simulink model "sampleModel84"  (R2021b)
settings: Solver=VariableStepAuto  StartTime=0.0  StopTime=10.0  RelTol=1e-3
undefined symbols (not defined in the file or in its folder): DiscIntNeverNeededParam, Newton, Raphson
libraries: simulink x7
settings Model: Creator=user  LastModifiedBy=user

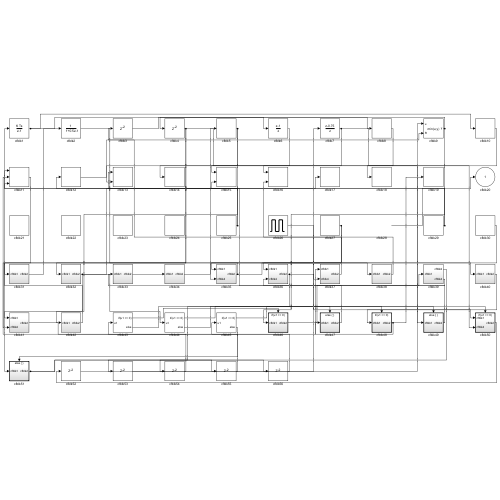
[thumbnail: Simulink's stored preview of the top-level diagram]
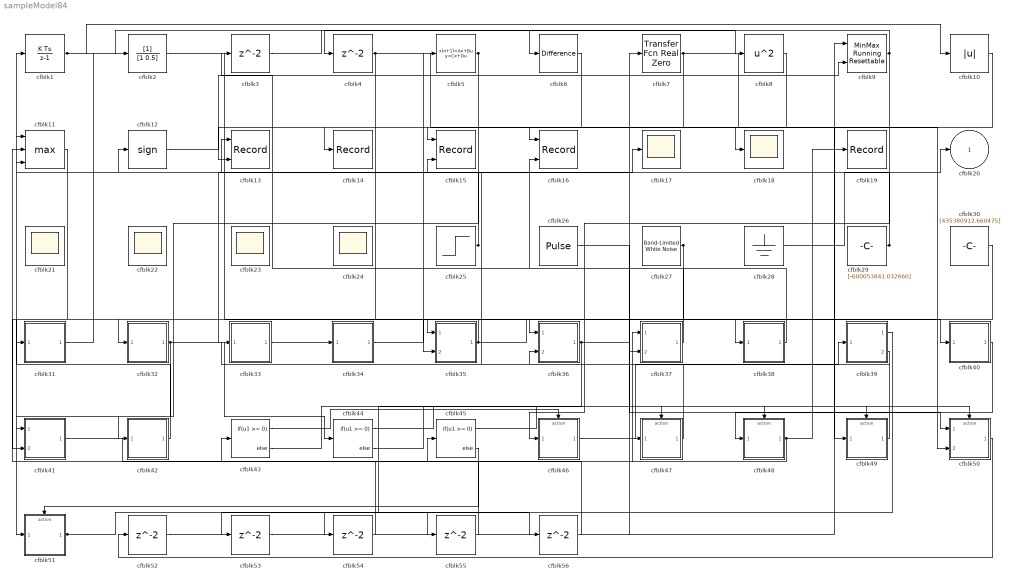
== system sampleModel84 ==
  cfblk1 : DiscreteIntegrator  ICPrevOutput=DiscIntNeverNeededParam  ICPrevScaledInput=DiscIntNeverNeededParam
  cfblk10 : Abs
  cfblk11 : MinMax  Function=max  Inputs=3
  cfblk12 : Signum
  cfblk13 : Record  FileSettingsInternal="{\"entries\":[{\"content\":{\"excelSettings\":{\"content\":{},\"type\":\"Streamout.ExcelSettings\"}},\"type\":\"Streamout.FileSettingStorage\",\"uuid\":\"6d5ab0e1-b9df-4df2-b804-9cd61c6ebc61\"}],\"packageUris\":[\"http://schema.mathworks.com/mf0/streamout_blocks/R2020a\"],\"version\":\"1.0\"}"  Layout=[1 1]  SignalsInternal="{\"entries\":[{\"content\":{\"signals\":[{\"content\":{\"blockPath\":[\"sampleModel84/cfblk13\"],\"channel\":[],\"dimensions\":[1],\"domain\":\"sampleModel84/cfblk13\",\"lineColor\":\"#a2142f\",\"plots\":[1],\"port\":1,\"sid\":[\"\"],\"signalID\":3042,\"signalName\":\"cfblk25\"},\"type\":\"RecordBlkView.Signal\",\"uuid\":\"d763d9ff-3473-40db-b6f0-cc00d4cb158e\"},{\"content\":{\"blockPath\":[\"sampleModel84/cfblk13\"],\"channel\":[],\"dimensions\":[1],\"domain\":\"sampleModel84/cfblk13\",\"lineColor\":\"#139fff\",\"plots\":[1],\"port\":2,\"sid\":[\"\"],\"signalID\":3046,\"signalName\":\"cfblk7\"},\"type\":\"RecordBlkView.Signal\",\"uuid\":\"d27f5f61-b032-4120-a613-3f0224b6e019\"}]},\"type\":\"RecordBlkView.InputSignals\",\"uuid\":\"3bd982ab-766d-439c-941a-6008472352c4\"}],\"packageUris\":[\"http://schema.mathworks.com/mf0/streamout_blocks/R2020a\"],\"version\":\"1.0\"}"  VisualizationBindings="{\"xyplotplugin\":{\"info\":[{\"series\":[{\"bindingParametersList\":[{\"parameter\":\"X-Axis\",\"signalID\":3042,\"signalName\":\"cfblk25\"},{\"parameter\":\"Y-Axis\",\"signalID\":3046,\"signalName\":\"cfblk7\"}],\"seriesID\":61716}],\"subplotID\":1}]}}"  CompatibilityTag=XY
  cfblk14 : Record  FileSettingsInternal="{\"entries\":[{\"content\":{\"excelSettings\":{\"content\":{},\"type\":\"Streamout.ExcelSettings\"}},\"type\":\"Streamout.FileSettingStorage\",\"uuid\":\"01d03471-c07e-448c-bcd4-e8026727b8ae\"}],\"packageUris\":[\"http://schema.mathworks.com/mf0/streamout_blocks/R2020a\"],\"version\":\"1.0\"}"  SignalsInternal="{\"entries\":[{\"content\":{\"signals\":[{\"content\":{\"blockPath\":[\"sampleModel84/cfblk14\"],\"channel\":[],\"dimensions\":[1],\"domain\":\"sampleModel84/cfblk14\",\"lineColor\":\"#a2142f\",\"plots\":[1],\"port\":1,\"sid\":[\"\"],\"signalID\":3050,\"signalName\":\"cfblk8\"},\"type\":\"RecordBlkView.Signal\",\"uuid\":\"eb13109a-bc49-49c4-8163-c11cf7b14920\"}]},\"type\":\"RecordBlkView.InputSignals\",\"uuid\":\"b3fcaa82-4256-42bf-8fc9-15e04aac9106\"}],\"packageUris\":[\"http://schema.mathworks.com/mf0/streamout_blocks/R2020a\"],\"version\":\"1.0\"}"  VisualizationBindings="{\"sparklinesplugin\":{\"info\":[{\"bindingParametersList\":[],\"subplotID\":1}]}}"
  cfblk15 : Record  FileSettingsInternal="{\"entries\":[{\"content\":{\"excelSettings\":{\"content\":{},\"type\":\"Streamout.ExcelSettings\"}},\"type\":\"Streamout.FileSettingStorage\",\"uuid\":\"8215706d-99e3-4ed1-b040-388dff8976c3\"}],\"packageUris\":[\"http://schema.mathworks.com/mf0/streamout_blocks/R2020a\"],\"version\":\"1.0\"}"  Layout=[1 1]  SignalsInternal="{\"entries\":[{\"content\":{\"signals\":[{\"content\":{\"blockPath\":[\"sampleModel84/cfblk15\"],\"channel\":[],\"dimensions\":[1],\"domain\":\"sampleModel84/cfblk15\",\"lineColor\":\"#a2142f\",\"plots\":[1],\"port\":1,\"sid\":[\"\"],\"signalID\":3054,\"signalName\":\"cfblk5\"},\"type\":\"RecordBlkView.Signal\",\"uuid\":\"c065fa96-9f8c-4313-8d4b-0e94634b5292\"},{\"content\":{\"blockPath\":[\"sampleModel84/cfblk15\"],\"channel\":[],\"dimensions\":[1],\"domain\":\"sampleModel84/cfblk15\",\"lineColor\":\"#139fff\",\"plots\":[1],\"port\":2,\"sid\":[\"\"],\"signalID\":3058,\"signalName\":\"cfblk49\"},\"type\":\"RecordBlkView.Signal\",\"uuid\":\"e4297feb-6ddb-4099-b980-2a59c267fa88\"}]},\"type\":\"RecordBlkView.InputSignals\",\"uuid\":\"14db0384-847c-431a-93a3-ba0fa706bc9d\"}],\"packageUris\":[\"http://schema.mathworks.com/mf0/streamout_blocks/R2020a\"],\"version\":\"1.0\"}"  VisualizationBindings="{\"xyplotplugin\":{\"info\":[{\"series\":[{\"bindingParametersList\":[{\"parameter\":\"X-Axis\",\"signalID\":3054,\"signalName\":\"cfblk5\"},{\"parameter\":\"Y-Axis\",\"signalID\":3058,\"signalName\":\"cfblk49\"}],\"seriesID\":40958}],\"subplotID\":1}]}}"  CompatibilityTag=XY
  cfblk16 : Record  FileSettingsInternal="{\"entries\":[{\"content\":{\"excelSettings\":{\"content\":{},\"type\":\"Streamout.ExcelSettings\"}},\"type\":\"Streamout.FileSettingStorage\",\"uuid\":\"8432e45c-109e-4b5d-958a-7ed43e91799e\"}],\"packageUris\":[\"http://schema.mathworks.com/mf0/streamout_blocks/R2020a\"],\"version\":\"1.0\"}"  Layout=[1 1]  SignalsInternal="{\"entries\":[{\"content\":{\"signals\":[{\"content\":{\"blockPath\":[\"sampleModel84/cfblk16\"],\"channel\":[],\"dimensions\":[1,1],\"domain\":\"sampleModel84/cfblk16\",\"lineColor\":\"#a2142f\",\"plots\":[1],\"port\":1,\"sid\":[\"\"],\"signalID\":3062,\"signalName\":\"cfblk6\"},\"type\":\"RecordBlkView.Signal\",\"uuid\":\"d31e46d2-4c50-47c9-b63a-65829e50d0df\"},{\"content\":{\"blockPath\":[\"sampleModel84/cfblk16\"],\"channel\":[],\"dimensions\":[1],\"domain\":\"sampleModel84/cfblk16\",\"lineColor\":\"#139fff\",\"plots\":[1],\"port\":2,\"sid\":[\"\"],\"signalID\":3066,\"signalName\":\"cfblk38\"},\"type\":\"RecordBlkView.Signal\",\"uuid\":\"c6a5d8c1-6799-48d2-840e-423a328fe3fe\"}]},\"type\":\"RecordBlkView.InputSignals\",\"uuid\":\"be483031-cf2c-4130-aa2f-949f5dc1496d\"}],\"packageUris\":[\"http://schema.mathworks.com/mf0/streamout_blocks/R2020a\"],\"version\":\"1.0\"}"  VisualizationBindings="{\"xyplotplugin\":{\"info\":[{\"series\":[{\"bindingParametersList\":[{\"parameter\":\"X-Axis\",\"signalID\":3062,\"signalName\":\"cfblk6\"},{\"parameter\":\"Y-Axis\",\"signalID\":3066,\"signalName\":\"cfblk38\"}],\"seriesID\":55547}],\"subplotID\":1}]}}"  CompatibilityTag=XY
  cfblk{17..18,21..24} (6 alike) : Scope
      cfblk21 settings: Floating=on
      cfblk22 settings: Floating=on
      cfblk23 settings: Floating=on
      cfblk24 settings: Floating=on
  cfblk19 : Record  FileSettingsInternal="{\"entries\":[{\"content\":{\"excelSettings\":{\"content\":{},\"type\":\"Streamout.ExcelSettings\"}},\"type\":\"Streamout.FileSettingStorage\",\"uuid\":\"b58bf4fe-9a4f-4d8d-a211-cbcb210b0c43\"}],\"packageUris\":[\"http://schema.mathworks.com/mf0/streamout_blocks/R2020a\"],\"version\":\"1.0\"}"  SignalsInternal="{\"entries\":[{\"content\":{\"signals\":[{\"content\":{\"blockPath\":[\"sampleModel84/cfblk19\"],\"channel\":[],\"dimensions\":[1,1],\"domain\":\"sampleModel84/cfblk19\",\"lineColor\":\"#ff13a6\",\"plots\":[1],\"port\":1,\"sid\":[\"\"],\"signalID\":3070,\"signalName\":\"cfblk48\"},\"type\":\"RecordBlkView.Signal\",\"uuid\":\"d2cc2008-ce60-42ec-8963-002263c80573\"}]},\"type\":\"RecordBlkView.InputSignals\",\"uuid\":\"16ff83b6-c59e-4d8c-a514-c0761e2915d2\"}],\"packageUris\":[\"http://schema.mathworks.com/mf0/streamout_blocks/R2020a\"],\"version\":\"1.0\"}"  VisualizationBindings="{\"sparklinesplugin\":{\"info\":[{\"bindingParametersList\":[],\"subplotID\":1}]}}"
  cfblk2 : DiscreteFilter  SampleTime=1
  cfblk25 : Step  Time=[41.000000]  Before=[-19914081.456809]  After=[534847659.507492]  SampleTime=0
  cfblk26 : DiscretePulseGenerator  PulseType=Time based  Amplitude=[-973417032.072928]  Period=[34845190.697167]  PulseWidth=5  PhaseDelay=[2.000000]
  cfblk27 : simulink/Sources/Band-Limited White Noise  Cov=[6295803502.230350]  Ts=0.1  seed=[3311985216.000000]
  cfblk28 : Ground
  cfblk29 : Constant  Value=[-600053841.032660]  SampleTime=1
  cfblk{3..4,52..56} (7 alike) : Delay  SampleTime=1
  cfblk30 : Constant  Value=[435380912.660475]  SampleTime=1
  cfblk31 : Subsystem
  cfblk32 : Subsystem
  cfblk33 : Subsystem
  cfblk34 : Subsystem
  cfblk35 : Subsystem
  cfblk36 : Subsystem
  cfblk37 : Subsystem
  cfblk38 : Subsystem
  cfblk39 : Subsystem
  cfblk40 : Subsystem
  cfblk41 : Subsystem
  cfblk42 : Subsystem
  cfblk43 : If  IfExpression=u1 >= 0  SampleTime=1
  cfblk44 : If  IfExpression=u1 >= 0  SampleTime=1
  cfblk45 : If  IfExpression=u1 >= 0  SampleTime=1
  cfblk46 : Subsystem  TreatAsAtomicUnit=on
  cfblk47 : Subsystem  TreatAsAtomicUnit=on
  cfblk48 : Subsystem  TreatAsAtomicUnit=on
  cfblk49 : Subsystem  TreatAsAtomicUnit=on
  cfblk5 : DiscreteStateSpace
  cfblk50 : Subsystem  TreatAsAtomicUnit=on
  cfblk51 : Subsystem  TreatAsAtomicUnit=on
  cfblk6 : simulink/Discrete/Difference  ICPrevInput=0.0  OutMin=[]  OutMax=[]  OutDataTypeStr=Inherit: Inherit via back propagation  OutDataType=fixdt(1, 16)  OutScaling=2^-10  DoSatur=off
  cfblk7 : simulink/Discrete/Transfer Fcn Real Zero  ZeroZ=0.75  ICPrevInput=0.0  DoSatur=off
      settings: SourceProductBaseCode=SL
  cfblk8 : Math  Operator=square  SaturateOnIntegerOverflow=on
  cfblk9 : simulink/Math Operations/MinMax Running Resettable  Function=min  vinit=0.0
  cfblk20 : Outport
  wires:
  cfblk5/1 -> cfblk15/1, cfblk42/1(cfblk1)
  cfblk9/1 -> cfblk4/1, cfblk46/1(cfblk1)
  cfblk40/1(cfblk2) -> cfblk48/1(cfblk1)
  cfblk51/1(cfblk2) -> cfblk55/1, cfblk56/1
  cfblk2/1 -> cfblk40/1(cfblk1)
  cfblk42/1(cfblk2) -> cfblk1/1
  cfblk48/1(cfblk2) -> cfblk37/1(cfblk1), cfblk19/1
  cfblk32/1(cfblk2) -> cfblk44/1, cfblk41/1(cfblk1), cfblk17/1
  cfblk46/1(cfblk2) -> cfblk39/1(cfblk1)
  cfblk6/1 -> cfblk16/1
  cfblk10/1 -> cfblk18/1
  cfblk3/1 -> cfblk6/1
  cfblk28/1 -> cfblk20/1
  cfblk31/1(cfblk2) -> cfblk2/1
  cfblk25/1 -> cfblk13/1, cfblk11/3
  cfblk30/1 -> cfblk36/1(cfblk1)
  cfblk27/1 -> cfblk35/1(cfblk1), cfblk35/2(cfblk4)
  cfblk7/1 -> cfblk13/2, cfblk50/2(cfblk4)
  cfblk35/1(cfblk2) -> cfblk32/1(cfblk1), cfblk38/1(cfblk1)
  cfblk33/1(cfblk2) -> cfblk34/1(cfblk1)
  cfblk26/1 -> cfblk37/2(cfblk4)
  cfblk1/1 -> cfblk10/1, cfblk8/1
  cfblk4/1 -> cfblk49/1(cfblk1), cfblk41/2(cfblk4), cfblk31/1(cfblk1)
  cfblk8/1 -> cfblk14/1
  cfblk47/1(cfblk2) -> cfblk33/1(cfblk1)
  cfblk39/2(cfblk4) -> cfblk36/2(cfblk4)
  cfblk34/1(cfblk2) -> cfblk5/1
  cfblk11/1 -> cfblk51/1(cfblk1)
  cfblk12/1 -> cfblk9/2
  cfblk29/1 -> cfblk12/1, cfblk11/1
  cfblk36/1(cfblk2) -> cfblk50/1(cfblk1), cfblk54/1
  cfblk49/1(cfblk2) -> cfblk15/2
  cfblk38/1(cfblk2) -> cfblk16/2
  cfblk37/1(cfblk2) -> cfblk3/1
  cfblk41/1(cfblk2) -> cfblk47/1(cfblk1)
  cfblk43/1 -> cfblk46/Action
  cfblk43/2 -> cfblk47/Action
  cfblk44/1 -> cfblk48/Action
  cfblk44/2 -> cfblk49/Action
  cfblk45/1 -> cfblk50/Action
  cfblk45/2 -> cfblk51/Action
  cfblk50/1(cfblk2) -> cfblk52/1
  cfblk52/1 -> cfblk7/1
  cfblk39/1(cfblk2) -> cfblk53/1
  cfblk53/1 -> cfblk9/1
  cfblk54/1 -> cfblk43/1
  cfblk55/1 -> cfblk45/1
  cfblk56/1 -> cfblk11/2

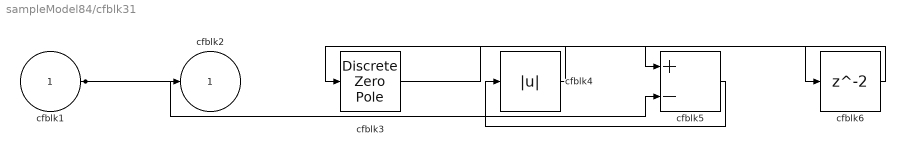
== system sampleModel84/cfblk31 ==
  cfblk1 : Inport
  cfblk3 : DiscreteZeroPole  Poles=[0 0.5]  Gain=1
  cfblk4 : Abs
  cfblk5 : Sum  Inputs=+-
  cfblk6 : Delay  SampleTime=1
  cfblk2 : Outport
  wires:
  cfblk4/1 -> cfblk3/1
  cfblk5/1 -> cfblk4/1
  cfblk1/1 -> cfblk5/2, cfblk2/1
  cfblk3/1 -> cfblk6/1
  cfblk6/1 -> cfblk5/1

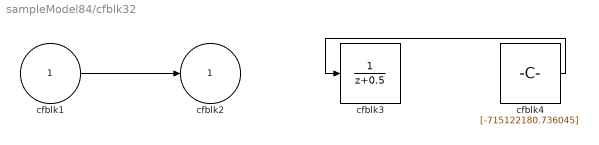
== system sampleModel84/cfblk32 ==
  cfblk1 : Inport
  cfblk3 : DiscreteTransferFcn  SampleTime=1
  cfblk4 : Constant  Value=[-715122180.736045]  SampleTime=1
  cfblk2 : Outport
  wires:
  cfblk4/1 -> cfblk3/1
  cfblk1/1 -> cfblk2/1

== system sampleModel84/cfblk33 ==
  cfblk1 : Inport
  cfblk3 : simulink/Discrete/Difference  ICPrevInput=0.0  OutMin=[]  OutMax=[]  OutDataTypeStr=Inherit: Inherit via back propagation  OutDataType=fixdt(1, 16)  OutScaling=2^-10  DoSatur=off
  cfblk2 : Outport
  wires:
  cfblk3/1 -> cfblk2/1
  cfblk1/1 -> cfblk3/1

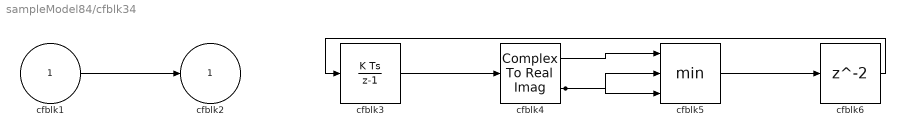
== system sampleModel84/cfblk34 ==
  cfblk1 : Inport
  cfblk3 : DiscreteIntegrator  ICPrevOutput=DiscIntNeverNeededParam  ICPrevScaledInput=DiscIntNeverNeededParam
  cfblk4 : ComplexToRealImag
  cfblk5 : MinMax  Inputs=3
  cfblk6 : Delay  SampleTime=1
  cfblk2 : Outport
  wires:
  cfblk1/1 -> cfblk2/1
  cfblk4/1 -> cfblk5/1
  cfblk3/1 -> cfblk4/1
  cfblk4/2 -> cfblk5/2, cfblk5/3
  cfblk5/1 -> cfblk6/1
  cfblk6/1 -> cfblk3/1

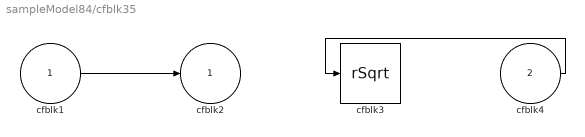
== system sampleModel84/cfblk35 ==
  cfblk1 : Inport
  cfblk4 : Inport  Port=2
  cfblk3 : Sqrt  Operator=rSqrt  AlgorithmType=Newton-Raphson  SaturateOnIntegerOverflow=on
  cfblk2 : Outport
  wires:
  cfblk4/1 -> cfblk3/1
  cfblk1/1 -> cfblk2/1

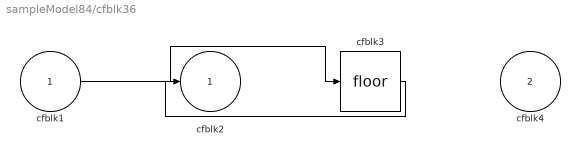
== system sampleModel84/cfblk36 ==
  cfblk1 : Inport
  cfblk4 : Inport  Port=2
  cfblk3 : Rounding
  cfblk2 : Outport
  wires:
  cfblk1/1 -> cfblk3/1
  cfblk3/1 -> cfblk2/1

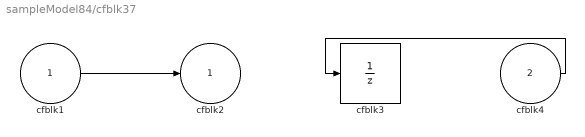
== system sampleModel84/cfblk37 ==
  cfblk1 : Inport
  cfblk4 : Inport  Port=2
  cfblk3 : UnitDelay  HasFrameUpgradeWarning=on
  cfblk2 : Outport
  wires:
  cfblk4/1 -> cfblk3/1
  cfblk1/1 -> cfblk2/1

== system sampleModel84/cfblk38 ==
  cfblk1 : Inport
  cfblk3 : Polyval  Coefs=[ +2.081618890e-019, -1.441693666e-014, +4.719686976e-010, -8.536869453e-006, +1.621573104e-001, -8.087801117e+001 ]
  cfblk2 : Outport
  wires:
  cfblk1/1 -> cfblk2/1, cfblk3/1

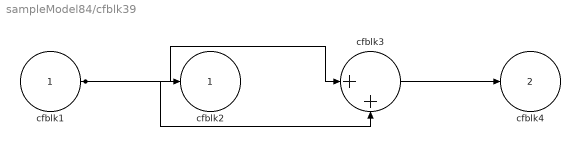
== system sampleModel84/cfblk39 ==
  cfblk1 : Inport
  cfblk3 : Sum  Inputs=|++
  cfblk2 : Outport
  cfblk4 : Outport  Port=2
  wires:
  cfblk1/1 -> cfblk3/1, cfblk2/1, cfblk3/2
  cfblk3/1 -> cfblk4/1

== system sampleModel84/cfblk40 ==
  cfblk1 : Inport
  cfblk3 : Constant  Value=[-783231984.092516]  SampleTime=1
  cfblk2 : Outport
  wires:
  cfblk1/1 -> cfblk2/1

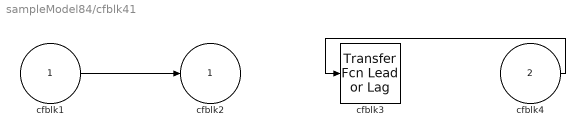
== system sampleModel84/cfblk41 ==
  cfblk1 : Inport
  cfblk4 : Inport  Port=2
  cfblk3 : simulink/Discrete/Transfer Fcn Lead or Lag  PoleZ=0.95  ZeroZ=0.75  ICPrevOutput=0.0  ICPrevInput=0.0  DoSatur=off
      settings: SourceProductBaseCode=SL
  cfblk2 : Outport
  wires:
  cfblk4/1 -> cfblk3/1
  cfblk1/1 -> cfblk2/1

== system sampleModel84/cfblk42 ==
  cfblk1 : Inport
  cfblk3 : DiscreteFir  SampleTime=1
  cfblk4 : Sin  TimeSource=Use external signal  SampleTime=0
  cfblk2 : Outport
  wires:
  cfblk1/1 -> cfblk3/1
  cfblk3/1 -> cfblk2/1, cfblk4/1

== system sampleModel84/cfblk46 ==
  cfblk1 : Inport
  Action Port : ActionPort  ActionPortLabel=if(u1 >= 0)
  cfblk3 : Sin  TimeSource=Use external signal  SampleTime=0
  cfblk2 : Outport
  wires:
  cfblk1/1 -> cfblk3/1
  cfblk3/1 -> cfblk2/1

== system sampleModel84/cfblk47 ==
  cfblk1 : Inport
  Action Port : ActionPort  ActionPortLabel=else
  cfblk3 : UnaryMinus
  cfblk2 : Outport
  wires:
  cfblk1/1 -> cfblk3/1
  cfblk3/1 -> cfblk2/1

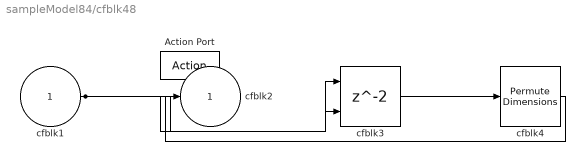
== system sampleModel84/cfblk48 ==
  cfblk1 : Inport
  Action Port : ActionPort  ActionPortLabel=if(u1 >= 0)
  cfblk3 : Delay  ShowEnablePort=on
      settings: InputPortMap=u0,e6
  cfblk4 : PermuteDimensions
  cfblk2 : Outport
  wires:
  cfblk3/1 -> cfblk4/1
  cfblk1/1 -> cfblk3/1, cfblk3/2
  cfblk4/1 -> cfblk2/1

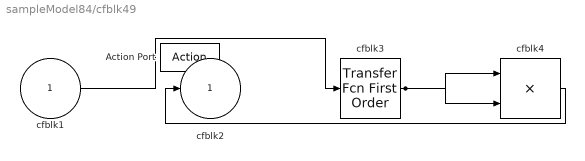
== system sampleModel84/cfblk49 ==
  cfblk1 : Inport
  Action Port : ActionPort  ActionPortLabel=else
  cfblk3 : simulink/Discrete/Transfer Fcn First Order  PoleZ=0.95  ICPrevOutput=0.0  DoSatur=off
  cfblk4 : Product
  cfblk2 : Outport
  wires:
  cfblk3/1 -> cfblk4/1, cfblk4/2
  cfblk4/1 -> cfblk2/1
  cfblk1/1 -> cfblk3/1

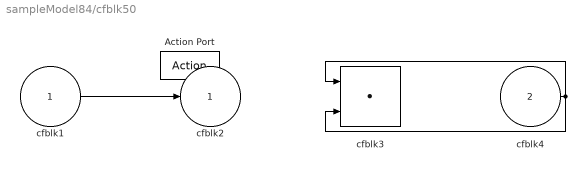
== system sampleModel84/cfblk50 ==
  cfblk1 : Inport
  cfblk4 : Inport  Port=2
  Action Port : ActionPort  ActionPortLabel=if(u1 >= 0)
  cfblk3 : DotProduct  InputSameDT=on  OutDataTypeStr=Inherit: Inherit via internal rule
  cfblk2 : Outport
  wires:
  cfblk1/1 -> cfblk2/1
  cfblk4/1 -> cfblk3/1, cfblk3/2

== system sampleModel84/cfblk51 ==
  cfblk1 : Inport
  Action Port : ActionPort  ActionPortLabel=else
  cfblk3 : ComplexToMagnitudeAngle
  cfblk2 : Outport
  wires:
  cfblk1/1 -> cfblk3/1
  cfblk3/1 -> cfblk2/1
